simulink model "SR26"  (R2025a)
settings: Solver=FixedStepDiscrete  StartTime=0.0  StopTime=100  FixedStep=0.01  RelTol=1e-3  EnableMultiTasking=on
PreLoadFcn:
  | try, model_open; catch, disp('Error occurred while executing model pre-load callback: model_open.m'); disp('Please assure that the MATLAB working directory is set to the model directory before opening.'); end
InitFcn:
  | try, model_open; catch, end
values from neighbouring files (symbols this model uses):
  dt = 10.0    [SR26.sldd]
undefined symbols (not defined in the file or in its folder): BMSInputProcessing, GCM, raptor_get_safe_string, raptor_xcp_function, RegenEnable, StateCAN, Subsystem, TCEnable
libraries: Utilities x263, Raptor_lib x137, simulink x7, IO x5, APPS_BSPC x4, TorqueCommand x3, Cooling x3, StateMachine x2, DriveSpeed x2, ATCC x2, BrakePressure x2, ThrottlePosition x2
(part 4 of 4)

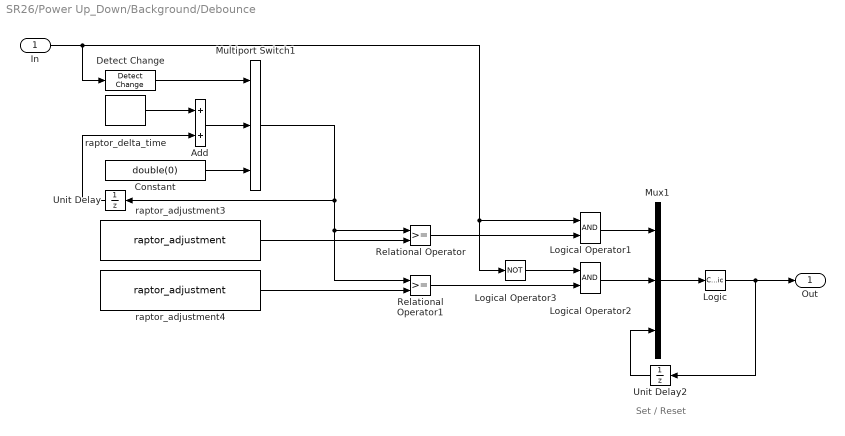
== system SR26/Power Up_Down/Background/Debounce ==
  note: Set / Reset
  In : Inport
  Add : Sum
  Constant : Constant  Value=double(0)
  Detect Change : simulink/Logic and Bit Operations/Detect Change  vinit=0  OutDataTypeStr=boolean
  Logic : CombinatorialLogic  TruthTable=[0;1;0;0;1;1;0;0]
  Logical Operator1 : Logic  AllPortsSameDT=off  OutDataTypeStr=boolean
  Logical Operator2 : Logic  AllPortsSameDT=off  OutDataTypeStr=boolean
  Logical Operator3 : Logic  Operator=NOT  Inputs=1  AllPortsSameDT=off  OutDataTypeStr=boolean
  Multiport Switch1 : MultiPortSwitch  DataPortOrder=Zero-based contiguous  Inputs=2  zeroidx=on  SaturateOnIntegerOverflow=off  InputSameDT=off
  Mux1 : Mux  Inputs=3
  Relational Operator : RelationalOperator  OutDataTypeStr=boolean  InputSameDT=off
  Relational Operator1 : RelationalOperator  OutDataTypeStr=boolean  InputSameDT=off
  Unit Delay : UnitDelay  SampleTime=-1  HasFrameUpgradeWarning=on
  Unit Delay2 : UnitDelay  InitialCondition=1  SampleTime=-1  HasFrameUpgradeWarning=on
  raptor_adjustment3 : Raptor_lib/Data Storage/raptor_adjustment  paramName='KeySwHiTimeThr'  nameSource=Parameter  initValue=0.2  dataType=double  storage=Calibration  calDispType=Number  calEnum={'Active Low', 'Active High'}  calGain=1  calOffset=0  calMax=inf  calMin=-inf  calFormat='-1'  calUnit='sec'  calHelp='State high time threshold'  calAccess=1  calFunction=group  calDispHeaders=off  calColHeaders={'Col1' 'Col2' 'Col3'}  calRowHeaders={'Row1' 'Row2' 'Row3'}
      settings: SourceProductName=Raptor
  raptor_adjustment4 : Raptor_lib/Data Storage/raptor_adjustment  paramName='KeySwLoTimeThr'  nameSource=Parameter  initValue=0.2  dataType=double  storage=Calibration  calDispType=Number  calEnum={'Active Low', 'Active High'}  calGain=1  calOffset=0  calMax=inf  calMin=-inf  calFormat='-1'  calUnit='sec'  calHelp='State low time threshold'  calAccess=1  calFunction=group  calDispHeaders=off  calColHeaders={'Col1' 'Col2' 'Col3'}  calRowHeaders={'Row1' 'Row2' 'Row3'}
      settings: SourceProductName=Raptor
  raptor_delta_time : Raptor_lib/Triggers/raptor_delta_time  unit=seconds
      settings: SourceProductName=Raptor
  Out : Outport  VectorParamsAs1DForOutWhenUnconnected=off
  wires:
  Detect Change/1 -> Multiport Switch1/1
  Logical Operator3/1 -> Logical Operator2/1
  Relational Operator/1 -> Logical Operator1/2
  Logical Operator2/1 -> Mux1/2
  Logical Operator1/1 -> Mux1/1
  Mux1/1 -> Logic/1
  Unit Delay2/1 -> Mux1/3
  In/1 -> Detect Change/1, Logical Operator1/1, Logical Operator3/1
  Multiport Switch1/1 -> Unit Delay/1, Relational Operator/1, Relational Operator1/1
  Add/1 -> Multiport Switch1/2
  Constant/1 -> Multiport Switch1/3
  Relational Operator1/1 -> Logical Operator2/2
  Logic/1 -> Unit Delay2/1, Out/1
  Unit Delay/1 -> Add/2
  raptor_delta_time/1 -> Add/1
  raptor_adjustment4/1 -> Relational Operator1/2
  raptor_adjustment3/1 -> Relational Operator/2

== system SR26/Power Up_Down/Background/Raise Shutdown Event ==
  Trigger : TriggerPort  TriggerType=falling  VariantControl=Variant
  Constant : Constant  Value=boolean(1)
  Function-Call Generator : FunctionCallGenerator  SampleTime=-1
  raptor_data_def : Raptor_lib/Data Storage/raptor_data_def  dataName='FgndTasksStopped'  initValue=0  dataType=boolean  storage=Volatile (RAM)  calVisible=on  calType=Measurement  calDispType=Number  calEnum={'False', 'True'}  calGain=1.0  calOffset=0  calMin=-Inf  calMax=Inf  calFormat='-1'  calUnit='Bool'  calHelp='Boolean indicating foreground tasks stopped'  calAccess=1  calFunction=group  calDispHeaders=off  calColHeaders={'Col1' 'Col2' 'Col3'}  calRowHeaders={'Row1' 'Row2' 'Row3'}
      settings: SourceProductName=Raptor
  raptor_data_write : Raptor_lib/Data Storage/raptor_data_write  dataName='FgndTasksStopped'  dataShape=Scalar  idxSource=Input Port  idxRow=1  idxCol=1
      settings: SourceProductName=Raptor
  raptor_shutdown : Raptor_lib/Triggers/raptor_shutdown  null=0
      settings: SourceProductName=Raptor
  wires:
  Constant/1 -> raptor_data_write/1
  Function-Call Generator/1 -> raptor_shutdown/Trigger

== system SR26/Power Up_Down/Background/Raise Startup Event ==
  Enable : EnablePort
  Trigger : TriggerPort  VariantControl=Variant
  Function-Call Generator : FunctionCallGenerator  SampleTime=-1
  raptor_startup : Raptor_lib/Triggers/raptor_startup  null=0
      settings: SourceProductName=Raptor
  wires:
  Function-Call Generator/1 -> raptor_startup/Trigger

== system SR26/Power Up_Down/Background/Store EEPROM ==
  Trigger : TriggerPort  TriggerType=falling  VariantControl=Variant
  Function-Call Generator : FunctionCallGenerator  SampleTime=-1
  raptor_store_nv : Raptor_lib/Data Storage/raptor_store_nv  null=0
      settings: SourceProductName=Raptor
  wires:
  Function-Call Generator/1 -> raptor_store_nv/Trigger

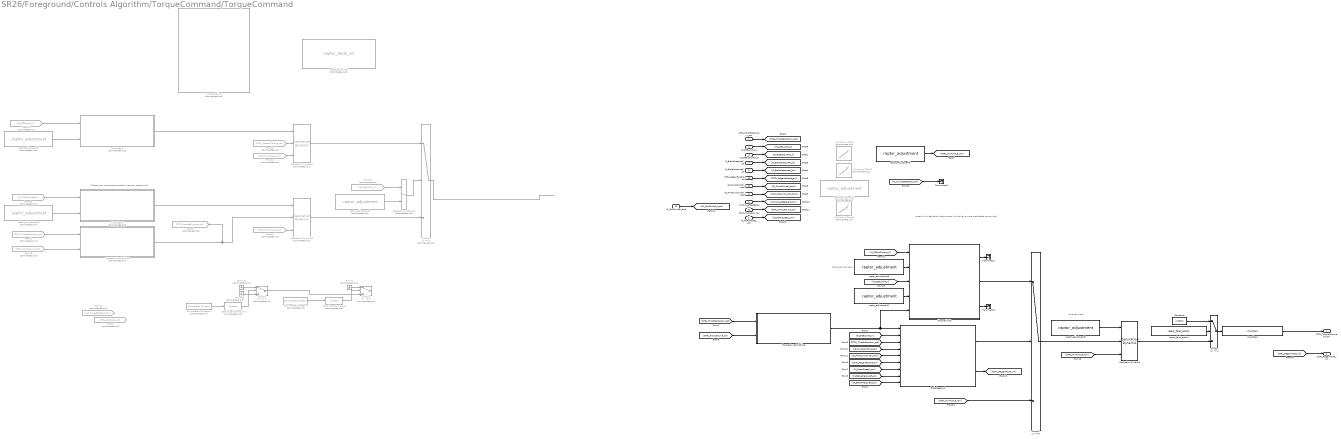
== system SR26/Foreground/Controls Algorithm/TorqueCommand/TorqueCommand ==
  note: current limit (set below legit current limit to have more predictable torque loss)
  note: hard cap here
  note: if there is an overcurrent condition, set new torque limit
  note: these are hard caps
  CTRL_ThrottlePosition_pct : Inport
  IN_DCBusVolt_V : Inport  Port=2
  IN_DCBusCurrent_A : Inport  Port=3
  IN_BrakePressureF_psi : Inport  Port=4
  IN_BrakePressureR_psi : Inport  Port=5
  IN_TorqueFeedback_Nm : Inport  Port=6
  IN_MotorSpeed_rpm : Inport  Port=7
  IO_PwrUpSwitch_bool : Inport  Port=8
  IO_PwrDownSwitch_bool : Inport  Port=9
  IO_CoolSwitch_bool : Inport  Port=10
  CTRL_TorqueCurve_en : Inport  Port=11
  CTRL_RegenEnable_en : Inport  Port=12
  1-D Lookup Table : Lookup_n-D  Commented=on  NumberOfTableDimensions=1  BreakpointsForDimension1=[0;50;100;120;130;140;150;160;170;180;190;200;205;210;215;220;225;230;235;240;245;250;255;260;265;270;275;280;285;290;295;300]  Table=[200;200;200;200;200;200;200;200;200;200;200;200;200;200;200;200;200;200;200;200;200;200;195;190;185;180;175;170;165;160;155;150]  InternalRulePriority=Speed  RndMeth=Simplest
  1-D Lookup Table1 : Lookup_n-D  Commented=on  NumberOfTableDimensions=1  BreakpointsForDimension1=[0;5;10;15;20;25;30;35;40;45;50;55;60;65;70;75;80;85;90;95;100]  Table=[0;3;6;9;12;15;25;35;45;55;65;75;85;95;105;115;135;155;175;195;200]  InternalRulePriority=Speed  RndMeth=Simplest
  1-D Lookup Table2 : Lookup_n-D  Commented=on  NumberOfTableDimensions=1  BreakpointsForDimension1=[0;100;200;205;210;215;220;225;230;235;240;245;250;255;260;265;270;275;280;285;290;300;310;320;330;400]  Table=[0;0;0;25;50;100;125;150;155;160;165;170;175;180;185;190;192;194;196;198;200;200;200;200;200;200]  InternalRulePriority=Speed  RndMeth=Simplest
  BrakeRegen_2 : Subsystem  AncestorBlock=TorqueCommand/BrakeRegen_2
  Constant1 : Constant  Value=uint8(0)
  Data Type Conversion : DataTypeConversion  Commented=on  OutDataTypeStr=boolean  SaturateOnIntegerOverflow=off  RndMeth=Floor
  Data Type Conversion1 : DataTypeConversion  Commented=on  OutDataTypeStr=boolean  SaturateOnIntegerOverflow=off  RndMeth=Floor
  Enumerated Constant : simulink/Sources/Enumerated Constant  Commented=on  OutDataTypeStr=Enum: RegenEnable  Value=RegenEnable.On  SampleTime=inf
  Enumerated Constant1 : simulink/Sources/Enumerated Constant  Commented=on  OutDataTypeStr=Enum: TCEnable  Value=TCEnable.On  SampleTime=inf
  From16 : From  Commented=on  GotoTag=IN_TorqueFeedback_Nm
  From23 : From  Commented=on  GotoTag=IN_DCBusVolt_V
  From24 : From  Commented=on  GotoTag=IN_DCBusVolt_V
  From25 : From  Commented=on  GotoTag=CTRL_AssistedTorque_Nm
  From26 : From  Commented=on  GotoTag=CTRL_MinTorque_Nm
  From27 : From  Commented=on  GotoTag=CTRL_ThrottlePosition_pct
  From28 : From  Commented=on  GotoTag=CTRL_MinTorque_Nm
  From29 : From  Commented=on  GotoTag=CTRL_TorqueCurve_en
  From30 : From  Commented=on  GotoTag=IN_DCBusCurrent_A
  From6 : From  Commented=on  GotoTag=CTRL_SlipRatio_na
  Goto14 : Goto  Commented=on  GotoTag=CTRL_AssistedTorque_Nm
  GreaterThanOrEqual2 : RelationalOperator  Commented=on  Operator=<=  OutDataTypeStr=boolean  RndMeth=Simplest  InputSameDT=off
  Ground : Ground  Commented=on
  Ground1 : Ground  Commented=on
  Ground2 : Ground  Commented=on
  OverMeas : Utilities/OverMeas  sigName='CTRL_TorqueCommand_Nm'  minimum=0  maximum=240
  Saturation Dynamic : simulink/Discontinuities/Saturation Dynamic  OutMin=[]  OutMax=[]  OutDataTypeStr=Inherit: Same as second input  OutDataType=fixdt(1, 16)  OutScaling=2^-10  DoSatur=off
  Saturation Dynamic3 : simulink/Discontinuities/Saturation Dynamic  Commented=on  OutMin=[]  OutMax=[]  OutDataTypeStr=Inherit: Same as second input  OutDataType=fixdt(1, 16)  OutScaling=2^-10  DoSatur=off
  Saturation Dynamic4 : simulink/Discontinuities/Saturation Dynamic  Commented=on  OutMin=[]  OutMax=[]  OutDataTypeStr=Inherit: Same as second input  OutDataType=fixdt(1, 16)  OutScaling=2^-10  DoSatur=off
  Subsystem2 : Subsystem  Commented=on
  Subsystem3 : Subsystem  Commented=on
  Switch : Switch  Criteria=u2 ~= 0  SaturateOnIntegerOverflow=off  InputSameDT=off
  Switch1 : Switch  Commented=on  Criteria=u2 ~= 0  OutDataTypeStr=single  SaturateOnIntegerOverflow=off  InputSameDT=off
  Switch2 : Switch  Criteria=u2 ~= 0  OutDataTypeStr=single  SaturateOnIntegerOverflow=off  InputSameDT=off
  Switch4 : Switch  Commented=on  Criteria=u2 ~= 0  SaturateOnIntegerOverflow=off  InputSameDT=off
  Switch5 : Switch  Commented=on  Criteria=u2 ~= 0  SaturateOnIntegerOverflow=off  InputSameDT=off
  Terminator1 : Terminator
  Terminator2 : Terminator
  Terminator3 : Terminator
  TorqueCeiling : Stateflow chart  Commented=on  TreatAsAtomicUnit=on
  TorqueCurveSwitching : Subsystem
  TorqueCurveSwitching1 : Subsystem  Commented=on
  TorqueLimits : Subsystem  AncestorBlock=TorqueCommand/TorqueLimits
  raptor_adjustment1 : Raptor_lib/Data Storage/raptor_adjustment  paramName='CTRL_DCBusUnderVoltThresh_V'  nameSource=Parameter  initValue=250  dataType=single  storage=Calibration  calDispType=Number  calEnum={'False', 'True'}  calGain=1.0  calOffset=0.0  calMax=378  calMin=-inf  calFormat='-1'  calUnit=''  calHelp=''  calAccess=1  calFunction=raptor_xcp_function(gcb)  calDispHeaders=off  calColHeaders={'Col1' 'Col2' 'Col3'}  calRowHeaders={'Row1' 'Row2' 'Row3'}
      settings: SourceProductName=Raptor
  raptor_adjustment10 : Raptor_lib/Data Storage/raptor_adjustment  Commented=on  paramName='CTRL_CurrentTorqueLimitSetting_na'  nameSource=Parameter  initValue=1  dataType=double  storage=Calibration  calDispType=Number  calEnum={'False', 'True'}  calGain=1.0  calOffset=0.0  calMax=3  calMin=1  calFormat='-1'  calUnit=''  calHelp=''  calAccess=1  calFunction=raptor_xcp_function(gcb)  calDispHeaders=off  calColHeaders={'Col1' 'Col2' 'Col3'}  calRowHeaders={'Row1' 'Row2' 'Row3'}
      settings: SourceProductName=Raptor
  raptor_adjustment11 : Raptor_lib/Data Storage/raptor_adjustment  Commented=on  paramName='CTRL_VoltageTorqueLimitSetting_Nm'  nameSource=Parameter  initValue=1  dataType=double  storage=Calibration  calDispType=Number  calEnum={'False', 'True'}  calGain=1.0  calOffset=0.0  calMax=3  calMin=1  calFormat='-1'  calUnit=''  calHelp=''  calAccess=1  calFunction=raptor_xcp_function(gcb)  calDispHeaders=off  calColHeaders={'Col1' 'Col2' 'Col3'}  calRowHeaders={'Row1' 'Row2' 'Row3'}
      settings: SourceProductName=Raptor
  raptor_adjustment2 : Raptor_lib/Data Storage/raptor_adjustment  paramName='CTRL_MaxTorque'  nameSource=Parameter  initValue=200  dataType=single  storage=Calibration  calDispType=Number  calEnum={'False', 'True'}  calGain=1.0  calOffset=0.0  calMax=230  calMin=0  calFormat='-1'  calUnit=''  calHelp=''  calAccess=1  calFunction=raptor_xcp_function(gcb)  calDispHeaders=off  calColHeaders={'Col1' 'Col2' 'Col3'}  calRowHeaders={'Row1' 'Row2' 'Row3'}
      settings: SourceProductName=Raptor
  raptor_adjustment3 : Raptor_lib/Data Storage/raptor_adjustment  Commented=on  paramName='CTRL_TorqueCurrLim_Nm'  nameSource=Parameter  initValue=100  dataType=single  storage=Calibration  calDispType=Number  calEnum={'False', 'True'}  calGain=1.0  calOffset=0.0  calMax=inf  calMin=-inf  calFormat='-1'  calUnit=''  calHelp=''  calAccess=1  calFunction=raptor_xcp_function(gcb)  calDispHeaders=off  calColHeaders={'Col1' 'Col2' 'Col3'}  calRowHeaders={'Row1' 'Row2' 'Row3'}
      settings: SourceProductName=Raptor
  raptor_adjustment5 : Raptor_lib/Data Storage/raptor_adjustment  paramName='CTRL_MinTorque'  nameSource=Parameter  initValue=-50  dataType=single  storage=Calibration  calDispType=Number  calEnum={'False', 'True'}  calGain=1.0  calOffset=0.0  calMax=230  calMin=-250  calFormat='-1'  calUnit=''  calHelp=''  calAccess=1  calFunction=raptor_xcp_function(gcb)  calDispHeaders=off  calColHeaders={'Col1' 'Col2' 'Col3'}  calRowHeaders={'Row1' 'Row2' 'Row3'}
      settings: SourceProductName=Raptor
  raptor_adjustment8 : Raptor_lib/Data Storage/raptor_adjustment  paramName='CTRL_DCBusOverCurrThresh_A'  nameSource=Parameter  initValue=140  dataType=single  storage=Calibration  calDispType=Number  calEnum={'False', 'True'}  calGain=1.0  calOffset=0.0  calMax=240  calMin=-inf  calFormat='-1'  calUnit=''  calHelp=''  calAccess=1  calFunction=raptor_xcp_function(gcb)  calDispHeaders=off  calColHeaders={'Col1' 'Col2' 'Col3'}  calRowHeaders={'Row1' 'Row2' 'Row3'}
      settings: SourceProductName=Raptor
  raptor_adjustment9 : Raptor_lib/Data Storage/raptor_adjustment  Commented=on  paramName='CTRL_DCBusUnderVoltThresh_V'  nameSource=Parameter  initValue=250  dataType=single  storage=Calibration  calDispType=Number  calEnum={'False', 'True'}  calGain=1.0  calOffset=0.0  calMax=240  calMin=-inf  calFormat='-1'  calUnit=''  calHelp=''  calAccess=1  calFunction=raptor_xcp_function(gcb)  calDispHeaders=off  calColHeaders={'Col1' 'Col2' 'Col3'}  calRowHeaders={'Row1' 'Row2' 'Row3'}
      settings: SourceProductName=Raptor
  raptor_fault_action : Raptor_lib/Faults/raptor_fault_action  actionName='TorqueCmdOverride'  calVisible=on  calAccess=1  calFunction='System | FaultManager | FaultAction'
      settings: SourceProductName=Raptor
  raptor_table_1d3 : Raptor_lib/Table Lookup/raptor_table_1d  Commented=on  dataName='CTRL_TargetSlipRatio_1D'  initValue=[0;764;1528;2293;3057;3822;4586;5350;6114;6880;7643]  dataType=single  storage=Calibration  initValueX=[12;12;12;12;12;12;11.5;11;10.5;10;8]  dataTypeXY=single  storageXY=Calibration  calVisible=on  showTable=on  calGain=1.0  calOffset=0.0  calMax=Inf  calMin=-Inf  calFormat='-1'  calUnit='pct'  calHelp=''  showBreakpoint=on  dataNameX=[]  calGainX=1.0  calOffsetX=0.0  calMaxX=Inf  calMinX=-Inf  calFormatX='-1'  calUnitX='rpm'  calHelpX=''  calAccess=1  calFunction=raptor_xcp_function(gcb)  measureEnable=off  mName=['Data1D_Output']
      settings: SourceProductName=Raptor
  CTRL_TorqueCommand_Nm : Outport
  CTRL_RegenMode_int : Outport  Port=2
  wires:
  TorqueLimits/1(CTRL_TorqueState_en) -> Terminator1/1
  [IN_DCBusVolt_V] -> TorqueLimits/3(IN_DCBusVoltage_V)
  TorqueCurveSwitching/1(Torque) -> BrakeRegen_2/1(TCTorque), TorqueLimits/5(CTRL_TorqueCurve_Nm)
  raptor_adjustment2/1 -> Saturation Dynamic/1
  TorqueLimits/2(CTRL_SafeTorqueCommand_Nm) -> Switch2/1
  [CTRL_MinTorque_Nm] -> Switch2/3
  Saturation Dynamic3/1 -> Switch1/3
  Subsystem2/1(CTRL_CurrentTorqueLimit_Nm) -> Saturation Dynamic3/1
  From24/1 -> Subsystem3/1(IN_DCBusVoltage_V)
  Subsystem3/1(CTRL_CurrentTorqueLimit_Nm) -> Saturation Dynamic4/1
  Saturation Dynamic4/1 -> Switch1/1
  GreaterThanOrEqual2/1 -> Switch1/2
  raptor_adjustment9/1 -> GreaterThanOrEqual2/2
  Switch1/1 -> ?
  From27/1 -> TorqueCurveSwitching1/1(CTRL_ThrottlePosition_pct)
  From29/1 -> TorqueCurveSwitching1/2(CTRL_TorqueCurve_en)
  From30/1 -> Subsystem2/1(IN_DCBusCurrent_A)
  From23/1 -> GreaterThanOrEqual2/1
  From25/1 -> Saturation Dynamic4/2
  From26/1 -> Saturation Dynamic4/3
  From28/1 -> Saturation Dynamic3/3
  raptor_adjustment10/1 -> Subsystem2/2(CTRL_CurrentTorqueSetting_na)
  raptor_adjustment11/1 -> Subsystem3/2(CTRL_VoltageTorqueSetting_na)
  TorqueCurveSwitching1/1(Torque) -> Goto14/1, Saturation Dynamic3/2
  raptor_adjustment8/1 -> TorqueLimits/2(CTRL_DCBusOverCurrThresh_A)
  raptor_adjustment1/1 -> TorqueLimits/4(CTRL_DCBusUnderVoltThresh_V)
  [IN_DCBusCurrent_A] -> TorqueLimits/1(IN_DCBusCurrent_A)
  IO_CoolSwitch_bool/1 -> [IO_CoolSwitch_bool]
  CTRL_TorqueCurve_en/1 -> [CTRL_TorqueCurve_en]
  [CTRL_MinTorque_Nm] -> Saturation Dynamic/3
  raptor_adjustment5/1 -> [CTRL_MinTorque_Nm]
  Ground2/1 -> Switch5/3
  Ground1/1 -> Switch5/1
  Data Type Conversion1/1 -> Switch5/2
  Data Type Conversion/1 -> Switch4/2
  Enumerated Constant1/1 -> Data Type Conversion1/1
  Enumerated Constant/1 -> Data Type Conversion/1
  Switch5/1 -> Switch4/3
  Ground/1 -> Switch4/1
  IN_TorqueFeedback_Nm/1 -> [IN_TorqueFeedback_Nm]
  IO_PwrUpSwitch_bool/1 -> [IO_PwrUpSwitch_bool]
  IO_PwrDownSwitch_bool/1 -> [IO_PwrDownSwitch_bool]
  [CTRL_TorqueCurve_en] -> TorqueCurveSwitching/2(CTRL_TorqueCurve_en)
  CTRL_RegenEnable_en/1 -> [CTRL_RegenEnable_en]
  IN_BrakePressureR_psi/1 -> [IN_BrakePressureR_psi]
  IN_BrakePressureF_psi/1 -> [IN_BrakePressureF_psi]
  CTRL_ThrottlePosition_pct/1 -> [CTRL_ThrottlePosition_pct]
  IN_DCBusCurrent_A/1 -> [IN_DCBusCurrent_A]
  IN_DCBusVolt_V/1 -> [IN_DCBusVolt_V]
  [CTRL_ThrottlePosition_pct] -> TorqueCurveSwitching/1(CTRL_ThrottlePosition_pct)
  Switch2/1 -> Saturation Dynamic/2
  Saturation Dynamic/1 -> Switch/3
  raptor_fault_action/1 -> Switch/2
  OverMeas/1 -> CTRL_TorqueCommand_Nm/1  "CTRL_TorqueCommand_Nm"
  Switch/1 -> OverMeas/1
  Constant1/1 -> Switch/1
  TorqueLimits/3(CTRL_TorqueRedux_Nm) -> Terminator2/1
  BrakeRegen_2/2(CTRL_RegenMode_int) -> [CTRL_RegenMode_int]
  [CTRL_RegenMode_int] -> CTRL_RegenMode_int/1
  [IN_TorqueFeedback_Nm] -> Terminator3/1
  IN_MotorSpeed_rpm/1 -> [IN_MotorSpeed_rpm]
  BrakeRegen_2/1(CTRL_RegenTorque_Nm) -> Switch2/2
  [CTRL_ThrottlePosition_pct] -> BrakeRegen_2/3(CTRL_ThrottlePosition_pct)
  [IN_DCBusVolt_V] -> BrakeRegen_2/2(IN_DCBusVolt_V)
  [IO_PwrUpSwitch_bool] -> BrakeRegen_2/4(IO_PwrUpSwitch_bool)
  [IO_PwrDownSwitch_bool] -> BrakeRegen_2/5(IO_PwrDownSwitch_bool)
  [CTRL_RegenEnable_en] -> BrakeRegen_2/6(CTRL_RegEnable_en)
  [IN_MotorSpeed_rpm] -> BrakeRegen_2/7(IN_MotorSpeed_rpm)
  [IN_BrakePressureF_psi] -> BrakeRegen_2/8(IN_BrakePressureF_psi)
  [IN_BrakePressureR_psi] -> BrakeRegen_2/9(IN_BrakePressureR_psi)

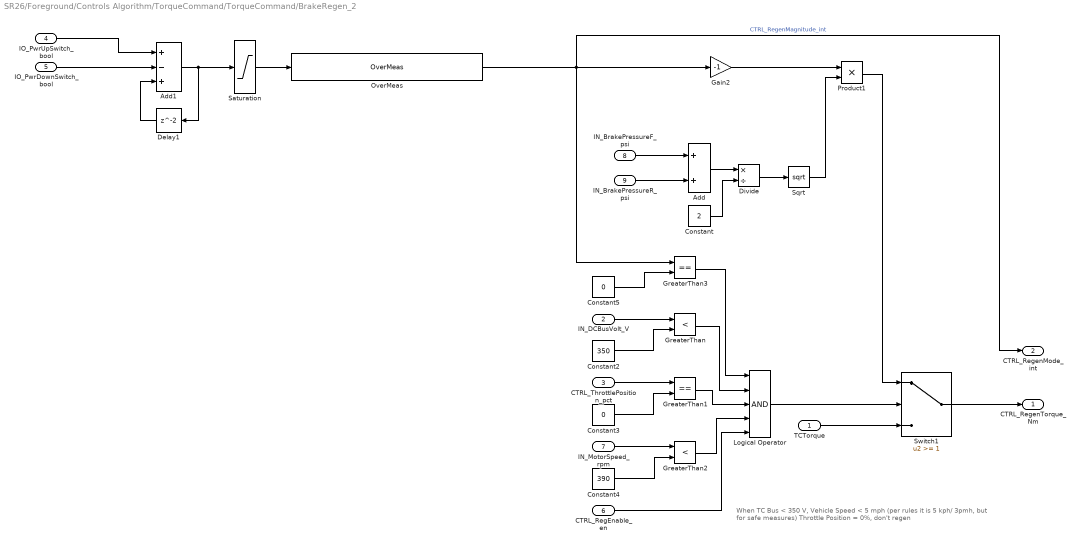
== system SR26/Foreground/Controls Algorithm/TorqueCommand/TorqueCommand/BrakeRegen_2 ==
  note: When TC Bus < 350 V,
      | Vehicle Speed < 5 mph (per rules it is 5 kph/ 3pmh, but for safe measures)
      | Throttle Position = 0%,
      | don't regen
  TCTorque : Inport
  IN_DCBusVolt_V : Inport  Port=2
  CTRL_ThrottlePosition_pct : Inport  Port=3
  IO_PwrUpSwitch_bool : Inport  Port=4
  IO_PwrDownSwitch_bool : Inport  Port=5
  CTRL_RegEnable_en : Inport  Port=6
  IN_MotorSpeed_rpm : Inport  Port=7
  IN_BrakePressureF_psi : Inport  Port=8
  IN_BrakePressureR_psi : Inport  Port=9
  Add : Sum
  Add1 : Sum  Inputs=+-+
  Constant : Constant  Value=2
  Constant2 : Constant  Value=350
  Constant3 : Constant  Value=0
  Constant4 : Constant  Value=390
  Constant5 : Constant  Value=0
  Delay1 : Delay
  Divide : Product  Inputs=*/
  Gain2 : Gain  Gain=-1
  GreaterThan : RelationalOperator  Operator=<  OutDataTypeStr=boolean  RndMeth=Simplest  InputSameDT=off
  GreaterThan1 : RelationalOperator  Operator===  OutDataTypeStr=boolean  RndMeth=Simplest  InputSameDT=off
  GreaterThan2 : RelationalOperator  Operator=<  OutDataTypeStr=boolean  RndMeth=Simplest  InputSameDT=off
  GreaterThan3 : RelationalOperator  Operator===  OutDataTypeStr=boolean  RndMeth=Simplest  InputSameDT=off
  Logical Operator : Logic  Inputs=5  AllPortsSameDT=off  OutDataTypeStr=boolean
  OverMeas : Utilities/OverMeas  sigName='CTRL_RegenMagnitude_int'  minimum=0  maximum=7
  Product1 : Product
  Saturation : Saturate  UpperLimit=7  LowerLimit=0
  Sqrt : Sqrt
  Switch1 : Switch  Threshold=1  SaturateOnIntegerOverflow=off  InputSameDT=off
  CTRL_RegenTorque_Nm : Outport
  CTRL_RegenMode_int : Outport  Port=2
  wires:
  Constant2/1 -> GreaterThan/2
  IN_DCBusVolt_V/1 -> GreaterThan/1
  CTRL_ThrottlePosition_pct/1 -> GreaterThan1/1
  Constant3/1 -> GreaterThan1/2
  IN_MotorSpeed_rpm/1 -> GreaterThan2/1
  Constant4/1 -> GreaterThan2/2
  Logical Operator/1 -> Switch1/2
  IO_PwrUpSwitch_bool/1 -> Add1/1
  IO_PwrDownSwitch_bool/1 -> Add1/2
  Add1/1 -> Saturation/1, Delay1/1
  Delay1/1 -> Add1/3
  Saturation/1 -> OverMeas/1
  TCTorque/1 -> Switch1/3
  OverMeas/1 -> GreaterThan3/1, CTRL_RegenMode_int/1, Gain2/1  "CTRL_RegenMagnitude_int"
  Constant5/1 -> GreaterThan3/2
  GreaterThan3/1 -> Logical Operator/1
  GreaterThan/1 -> Logical Operator/2
  GreaterThan1/1 -> Logical Operator/3
  GreaterThan2/1 -> Logical Operator/4
  CTRL_RegEnable_en/1 -> Logical Operator/5
  Sqrt/1 -> Product1/2
  Divide/1 -> Sqrt/1
  IN_BrakePressureF_psi/1 -> Add/1
  Add/1 -> Divide/1
  Constant/1 -> Divide/2
  IN_BrakePressureR_psi/1 -> Add/2
  Gain2/1 -> Product1/1
  Product1/1 -> Switch1/1
  Switch1/1 -> CTRL_RegenTorque_Nm/1

== system SR26/Foreground/Controls Algorithm/TorqueCommand/TorqueCommand/Subsystem2 ==
  note: decrease at 180A
  note: decrease at 180A
  note: decrease at 150A
  IN_DCBusCurrent_A : Inport
  CTRL_CurrentTorqueSetting_na : Inport  Port=2
  Multiport Switch : MultiPortSwitch  SaturateOnIntegerOverflow=off  InputSameDT=off
  raptor_table_1d1 : Raptor_lib/Table Lookup/raptor_table_1d  dataName='CTRL_CurrentToLimTorqueCmd2_1D'  initValue=[230;230;226;214;194;166;130;86;34;0]  dataType=single  storage=Calibration  initValueX=[0;180;190;200;210;220;230;240;250;260]  dataTypeXY=single  storageXY=Calibration  calVisible=on  showTable=on  calGain=1.0  calOffset=0.0  calMax=Inf  calMin=-Inf  calFormat='-1'  calUnit='Nm'  calHelp=''  showBreakpoint=on  dataNameX=[]  calGainX=1.0  calOffsetX=0.0  calMaxX=Inf  calMinX=-Inf  calFormatX='-1'  calUnitX='A'  calHelpX=''  calAccess=1  calFunction=raptor_xcp_function(gcb)  measureEnable=off  mName=['Data1D_Output']
      settings: SourceProductName=Raptor
  raptor_table_1d2 : Raptor_lib/Table Lookup/raptor_table_1d  dataName='CTRL_CurrentToLimTorqueCmd_1D'  initValue=[230;228;226;222;218;212;206;198;190;180;170;158;146;132;118;102;86;68;50;30;10;0]  dataType=single  storage=Calibration  initValueX=[0;150;155;160;165;170;175;180;185;190;195;200;205;210;215;220;225;230;235;240;245;250]  dataTypeXY=single  storageXY=Calibration  calVisible=on  showTable=on  calGain=1.0  calOffset=0.0  calMax=Inf  calMin=-Inf  calFormat='-1'  calUnit='Nm'  calHelp=''  showBreakpoint=on  dataNameX=[]  calGainX=1.0  calOffsetX=0.0  calMaxX=Inf  calMinX=-Inf  calFormatX='-1'  calUnitX='A'  calHelpX=''  calAccess=1  calFunction=raptor_xcp_function(gcb)  measureEnable=off  mName=['Data1D_Output']
      settings: SourceProductName=Raptor
  raptor_table_1d3 : Raptor_lib/Table Lookup/raptor_table_1d  dataName='CTRL_CurrentToLimTorqueCmd3_1D'  initValue=[230;230;226;214;194;166;130;86;34;0]  dataType=single  storage=Calibration  initValueX=[0;150;160;170;180;190;200;210;220;230]  dataTypeXY=single  storageXY=Calibration  calVisible=on  showTable=on  calGain=1.0  calOffset=0.0  calMax=Inf  calMin=-Inf  calFormat='-1'  calUnit='Nm'  calHelp=''  showBreakpoint=on  dataNameX=[]  calGainX=1.0  calOffsetX=0.0  calMaxX=Inf  calMinX=-Inf  calFormatX='-1'  calUnitX='A'  calHelpX=''  calAccess=1  calFunction=raptor_xcp_function(gcb)  measureEnable=off  mName=['Data1D_Output']
      settings: SourceProductName=Raptor
  CTRL_CurrentTorqueLimit_Nm : Outport
  wires:
  CTRL_CurrentTorqueSetting_na/1 -> Multiport Switch/1
  raptor_table_1d2/1 -> Multiport Switch/2
  raptor_table_1d1/1 -> Multiport Switch/3
  raptor_table_1d3/1 -> Multiport Switch/4
  IN_DCBusCurrent_A/1 -> raptor_table_1d3/1, raptor_table_1d1/1, raptor_table_1d2/1
  Multiport Switch/1 -> CTRL_CurrentTorqueLimit_Nm/1

== system SR26/Foreground/Controls Algorithm/TorqueCommand/TorqueCommand/Subsystem3 ==
  IN_DCBusVoltage_V : Inport
  CTRL_VoltageTorqueSetting_na : Inport  Port=2
  Multiport Switch : MultiPortSwitch  SaturateOnIntegerOverflow=off  InputSameDT=off
  raptor_table_1d1 : Raptor_lib/Table Lookup/raptor_table_1d  dataName='CTRL_VoltageToLimTorqueCmd2_1D'  initValue=[0;0;230;230]  dataType=double  storage=Calibration  initValueX=[0;225;280;378]  dataTypeXY=double  storageXY=Calibration  calVisible=on  showTable=on  calGain=1.0  calOffset=0.0  calMax=Inf  calMin=-Inf  calFormat='-1'  calUnit='Nm'  calHelp=''  showBreakpoint=on  dataNameX=[]  calGainX=1.0  calOffsetX=0.0  calMaxX=Inf  calMinX=-Inf  calFormatX='-1'  calUnitX='V'  calHelpX=''  calAccess=1  calFunction=raptor_xcp_function(gcb)  measureEnable=off  mName=['Data1D_Output']
      settings: SourceProductName=Raptor
  raptor_table_1d2 : Raptor_lib/Table Lookup/raptor_table_1d  dataName='CTRL_VoltageToLimTorqueCmd_1D'  initValue=[0;0;230;230]  dataType=double  storage=Calibration  initValueX=[0;225;280;378]  dataTypeXY=double  storageXY=Calibration  calVisible=on  showTable=on  calGain=1.0  calOffset=0.0  calMax=Inf  calMin=-Inf  calFormat='-1'  calUnit='Nm'  calHelp=''  showBreakpoint=on  dataNameX=[]  calGainX=1.0  calOffsetX=0.0  calMaxX=Inf  calMinX=-Inf  calFormatX='-1'  calUnitX='V'  calHelpX=''  calAccess=1  calFunction=raptor_xcp_function(gcb)  measureEnable=off  mName=['Data1D_Output']
      settings: SourceProductName=Raptor
  raptor_table_1d3 : Raptor_lib/Table Lookup/raptor_table_1d  dataName='CTRL_VoltageToLimTorqueCmd3_1D'  initValue=[0;0;230;230]  dataType=double  storage=Calibration  initValueX=[0;225;280;378]  dataTypeXY=double  storageXY=Calibration  calVisible=on  showTable=on  calGain=1.0  calOffset=0.0  calMax=Inf  calMin=-Inf  calFormat='-1'  calUnit='Nm'  calHelp=''  showBreakpoint=on  dataNameX=[]  calGainX=1.0  calOffsetX=0.0  calMaxX=Inf  calMinX=-Inf  calFormatX='-1'  calUnitX='V'  calHelpX=''  calAccess=1  calFunction=raptor_xcp_function(gcb)  measureEnable=off  mName=['Data1D_Output']
      settings: SourceProductName=Raptor
  CTRL_CurrentTorqueLimit_Nm : Outport
  wires:
  Multiport Switch/1 -> CTRL_CurrentTorqueLimit_Nm/1
  IN_DCBusVoltage_V/1 -> raptor_table_1d2/1, raptor_table_1d3/1, raptor_table_1d1/1
  raptor_table_1d3/1 -> Multiport Switch/4
  raptor_table_1d1/1 -> Multiport Switch/3
  raptor_table_1d2/1 -> Multiport Switch/2
  CTRL_VoltageTorqueSetting_na/1 -> Multiport Switch/1

== system SR26/Foreground/Controls Algorithm/TorqueCommand/TorqueCommand/TorqueCurveSwitching ==
  CTRL_ThrottlePosition_pct : Inport
  CTRL_TorqueCurve_en : Inport  Port=2
  Add : Sum
  Carter : Raptor_lib/Table Lookup/raptor_table_1d  dataName='CTRL_ThrottleToTorqueCmdCarter_1D'  initValue=[0;1;3;6;11;18;25;34;45;57;70;85;101;118;137;158;179;202;227;230;230]  dataType=single  storage=Calibration  initValueX=[0;5;10;15;20;25;30;35;40;45;50;55;60;65;70;75;80;85;90;95;100]  dataTypeXY=single  storageXY=Calibration  calVisible=on  showTable=on  calGain=1.0  calOffset=0.0  calMax=Inf  calMin=-Inf  calFormat='-1'  calUnit='pct'  calHelp=''  showBreakpoint=on  dataNameX=[]  calGainX=1.0  calOffsetX=0.0  calMaxX=Inf  calMinX=-Inf  calFormatX='-1'  calUnitX='Nm'  calHelpX=''  calAccess=1  calFunction=raptor_xcp_function(gcb)  measureEnable=off  mName=['Data1D_Output']
      settings: SourceProductName=Raptor
  Casey : Raptor_lib/Table Lookup/raptor_table_1d  dataName='CTRL_ThrottleToTorqueCmdCasey_1D'  initValue=[0;3;6;9;12;15;25;35;45;55;65;75;85;95;105;115;135;155;175;195;200]  dataType=single  storage=Calibration  initValueX=[0;5;10;15;20;25;30;35;40;45;50;55;60;65;70;75;80;85;90;95;100]  dataTypeXY=single  storageXY=Calibration  calVisible=on  showTable=on  calGain=1.0  calOffset=0.0  calMax=Inf  calMin=-Inf  calFormat='-1'  calUnit='pct'  calHelp=''  showBreakpoint=on  dataNameX=[]  calGainX=1.0  calOffsetX=0.0  calMaxX=Inf  calMinX=-Inf  calFormatX='-1'  calUnitX='Nm'  calHelpX=''  calAccess=1  calFunction=raptor_xcp_function(gcb)  measureEnable=off  mName=['Data1D_Output']
      settings: SourceProductName=Raptor
  Constant : Constant
  Data Type Conversion : DataTypeConversion  OutDataTypeStr=uint8  SaturateOnIntegerOverflow=off  RndMeth=Floor
  Default : Raptor_lib/Table Lookup/raptor_table_1d  dataName='CTRL_ThrottleToTorqueCmdDef_1D'  initValue=[0;3;6;9;12;15;25;35;45;55;65;75;85;95;105;115;135;155;175;195;200]  dataType=single  storage=Calibration  initValueX=[0;5;10;15;20;25;30;35;40;45;50;55;60;65;70;75;80;85;90;95;100]  dataTypeXY=single  storageXY=Calibration  calVisible=on  showTable=on  calGain=1.0  calOffset=0.0  calMax=Inf  calMin=-Inf  calFormat='-1'  calUnit='pct'  calHelp=''  showBreakpoint=on  dataNameX=[]  calGainX=1.0  calOffsetX=0.0  calMaxX=Inf  calMinX=-Inf  calFormatX='-1'  calUnitX='Nm'  calHelpX=''  calAccess=1  calFunction=raptor_xcp_function(gcb)  measureEnable=off  mName=['Data1D_Output']
      settings: SourceProductName=Raptor
  Lim100 : Raptor_lib/Table Lookup/raptor_table_1d  dataName='CTRL_ThrottleToTorqueCmd100_1D'  initValue=[0;8;17;25;33;40;48;55;62;68;74;79;84;88;92;95;97;99;100;100;100]  dataType=single  storage=Calibration  initValueX=[0;5;10;15;20;25;30;35;40;45;50;55;60;65;70;75;80;85;90;95;100]  dataTypeXY=single  storageXY=Calibration  calVisible=on  showTable=on  calGain=1.0  calOffset=0.0  calMax=Inf  calMin=-Inf  calFormat='-1'  calUnit='pct'  calHelp=''  showBreakpoint=on  dataNameX=[]  calGainX=1.0  calOffsetX=0.0  calMaxX=Inf  calMinX=-Inf  calFormatX='-1'  calUnitX='Nm'  calHelpX=''  calAccess=1  calFunction=raptor_xcp_function(gcb)  measureEnable=off  mName=['Data1D_Output']
      settings: SourceProductName=Raptor
  Lim150 : Raptor_lib/Table Lookup/raptor_table_1d  dataName='CTRL_ThrottleToTorqueCmd150_1D'  initValue=[0;8;17;25;33;40;48;55;62;68;74;79;84;88;92;95;97;99;100;100;100]  dataType=single  storage=Calibration  initValueX=[0;5;10;15;20;25;30;35;40;45;50;55;60;65;70;75;80;85;90;95;100]  dataTypeXY=single  storageXY=Calibration  calVisible=on  showTable=on  calGain=1.0  calOffset=0.0  calMax=Inf  calMin=-Inf  calFormat='-1'  calUnit='pct'  calHelp=''  showBreakpoint=on  dataNameX=[]  calGainX=1.0  calOffsetX=0.0  calMaxX=Inf  calMinX=-Inf  calFormatX='-1'  calUnitX='Nm'  calHelpX=''  calAccess=1  calFunction=raptor_xcp_function(gcb)  measureEnable=off  mName=['Data1D_Output']
      settings: SourceProductName=Raptor
  Matt : Raptor_lib/Table Lookup/raptor_table_1d  dataName='CTRL_ThrottleToTorqueCmdMatt_1D'  initValue=[0;3;6;9;12;15;25;35;45;55;65;75;85;95;105;115;135;155;175;195;200]  dataType=single  storage=Calibration  initValueX=[0;5;10;15;20;25;30;35;40;45;50;55;60;65;70;75;80;85;90;95;100]  dataTypeXY=single  storageXY=Calibration  calVisible=on  showTable=on  calGain=1.0  calOffset=0.0  calMax=Inf  calMin=-Inf  calFormat='-1'  calUnit='pct'  calHelp=''  showBreakpoint=on  dataNameX=[]  calGainX=1.0  calOffsetX=0.0  calMaxX=Inf  calMinX=-Inf  calFormatX='-1'  calUnitX='Nm'  calHelpX=''  calAccess=1  calFunction=raptor_xcp_function(gcb)  measureEnable=off  mName=['Data1D_Output']
      settings: SourceProductName=Raptor
  Multiport Switch : MultiPortSwitch  Inputs=7  SaturateOnIntegerOverflow=off  InputSameDT=off
  Noah : Raptor_lib/Table Lookup/raptor_table_1d  dataName='CTRL_ThrottleToTorqueCmdNoah_1D'  initValue=[0;3;6;9;12;15;25;35;45;55;65;75;85;95;105;115;135;155;175;195;200]  dataType=single  storage=Calibration  initValueX=[0;5;10;15;20;25;30;35;40;45;50;55;60;65;70;75;80;85;90;95;100]  dataTypeXY=single  storageXY=Calibration  calVisible=on  showTable=on  calGain=1.0  calOffset=0.0  calMax=Inf  calMin=-Inf  calFormat='-1'  calUnit='pct'  calHelp=''  showBreakpoint=on  dataNameX=[]  calGainX=1.0  calOffsetX=0.0  calMaxX=Inf  calMinX=-Inf  calFormatX='-1'  calUnitX='Nm'  calHelpX=''  calAccess=1  calFunction=raptor_xcp_function(gcb)  measureEnable=off  mName=['Data1D_Output']
      settings: SourceProductName=Raptor
  Torque : Outport
  wires:
  Data Type Conversion/1 -> Add/1
  Constant/1 -> Add/2
  Add/1 -> Multiport Switch/1
  CTRL_TorqueCurve_en/1 -> Data Type Conversion/1
  Multiport Switch/1 -> Torque/1
  Lim100/1 -> Multiport Switch/8
  Lim150/1 -> Multiport Switch/7
  Carter/1 -> Multiport Switch/6
  Noah/1 -> Multiport Switch/5
  Casey/1 -> Multiport Switch/4
  Matt/1 -> Multiport Switch/3
  Default/1 -> Multiport Switch/2
  CTRL_ThrottlePosition_pct/1 -> Matt/1, Casey/1, Noah/1, Carter/1, Lim100/1, Lim150/1, Default/1  "100Nm Limit"

== system SR26/Foreground/Controls Algorithm/TorqueCommand/TorqueCommand/TorqueCurveSwitching1 ==
  CTRL_ThrottlePosition_pct : Inport
  CTRL_TorqueCurve_en : Inport  Port=2
  Add : Sum
  Carter : Raptor_lib/Table Lookup/raptor_table_1d  dataName='CTRL_ThrottleToTorqueCmdCarter_1D'  initValue=[0;1;3;6;11;18;25;34;45;57;70;85;101;118;137;158;179;202;227;230;230]  dataType=single  storage=Calibration  initValueX=[0;5;10;15;20;25;30;35;40;45;50;55;60;65;70;75;80;85;90;95;100]  dataTypeXY=single  storageXY=Calibration  calVisible=on  showTable=on  calGain=1.0  calOffset=0.0  calMax=Inf  calMin=-Inf  calFormat='-1'  calUnit='pct'  calHelp=''  showBreakpoint=on  dataNameX=[]  calGainX=1.0  calOffsetX=0.0  calMaxX=Inf  calMinX=-Inf  calFormatX='-1'  calUnitX='Nm'  calHelpX=''  calAccess=1  calFunction=raptor_xcp_function(gcb)  measureEnable=off  mName=['Data1D_Output']
      settings: SourceProductName=Raptor
  Casey : Raptor_lib/Table Lookup/raptor_table_1d  dataName='CTRL_ThrottleToTorqueCmdCasey_1D'  initValue=[0;3;6;9;12;15;25;35;45;55;65;75;85;95;105;115;135;155;175;195;200]  dataType=single  storage=Calibration  initValueX=[0;5;10;15;20;25;30;35;40;45;50;55;60;65;70;75;80;85;90;95;100]  dataTypeXY=single  storageXY=Calibration  calVisible=on  showTable=on  calGain=1.0  calOffset=0.0  calMax=Inf  calMin=-Inf  calFormat='-1'  calUnit='pct'  calHelp=''  showBreakpoint=on  dataNameX=[]  calGainX=1.0  calOffsetX=0.0  calMaxX=Inf  calMinX=-Inf  calFormatX='-1'  calUnitX='Nm'  calHelpX=''  calAccess=1  calFunction=raptor_xcp_function(gcb)  measureEnable=off  mName=['Data1D_Output']
      settings: SourceProductName=Raptor
  Constant : Constant
  Data Type Conversion : DataTypeConversion  OutDataTypeStr=uint8  SaturateOnIntegerOverflow=off  RndMeth=Floor
  Default : Raptor_lib/Table Lookup/raptor_table_1d  dataName='CTRL_ThrottleToTorqueCmdDef_1D'  initValue=[0;3;6;9;12;15;25;35;45;55;65;75;85;95;105;115;135;155;175;195;200]  dataType=single  storage=Calibration  initValueX=[0;5;10;15;20;25;30;35;40;45;50;55;60;65;70;75;80;85;90;95;100]  dataTypeXY=single  storageXY=Calibration  calVisible=on  showTable=on  calGain=1.0  calOffset=0.0  calMax=Inf  calMin=-Inf  calFormat='-1'  calUnit='pct'  calHelp=''  showBreakpoint=on  dataNameX=[]  calGainX=1.0  calOffsetX=0.0  calMaxX=Inf  calMinX=-Inf  calFormatX='-1'  calUnitX='Nm'  calHelpX=''  calAccess=1  calFunction=raptor_xcp_function(gcb)  measureEnable=off  mName=['Data1D_Output']
      settings: SourceProductName=Raptor
  Lim100 : Raptor_lib/Table Lookup/raptor_table_1d  dataName='CTRL_ThrottleToTorqueCmd100_1D'  initValue=[0;8;17;25;33;40;48;55;62;68;74;79;84;88;92;95;97;99;100;100;100]  dataType=single  storage=Calibration  initValueX=[0;5;10;15;20;25;30;35;40;45;50;55;60;65;70;75;80;85;90;95;100]  dataTypeXY=single  storageXY=Calibration  calVisible=on  showTable=on  calGain=1.0  calOffset=0.0  calMax=Inf  calMin=-Inf  calFormat='-1'  calUnit='pct'  calHelp=''  showBreakpoint=on  dataNameX=[]  calGainX=1.0  calOffsetX=0.0  calMaxX=Inf  calMinX=-Inf  calFormatX='-1'  calUnitX='Nm'  calHelpX=''  calAccess=1  calFunction=raptor_xcp_function(gcb)  measureEnable=off  mName=['Data1D_Output']
      settings: SourceProductName=Raptor
  Lim150 : Raptor_lib/Table Lookup/raptor_table_1d  dataName='CTRL_ThrottleToTorqueCmd150_1D'  initValue=[0;8;17;25;33;40;48;55;62;68;74;79;84;88;92;95;97;99;100;100;100]  dataType=single  storage=Calibration  initValueX=[0;5;10;15;20;25;30;35;40;45;50;55;60;65;70;75;80;85;90;95;100]  dataTypeXY=single  storageXY=Calibration  calVisible=on  showTable=on  calGain=1.0  calOffset=0.0  calMax=Inf  calMin=-Inf  calFormat='-1'  calUnit='pct'  calHelp=''  showBreakpoint=on  dataNameX=[]  calGainX=1.0  calOffsetX=0.0  calMaxX=Inf  calMinX=-Inf  calFormatX='-1'  calUnitX='Nm'  calHelpX=''  calAccess=1  calFunction=raptor_xcp_function(gcb)  measureEnable=off  mName=['Data1D_Output']
      settings: SourceProductName=Raptor
  Matt : Raptor_lib/Table Lookup/raptor_table_1d  dataName='CTRL_ThrottleToTorqueCmdMatt_1D'  initValue=[0;3;6;9;12;15;25;35;45;55;65;75;85;95;105;115;135;155;175;195;200]  dataType=single  storage=Calibration  initValueX=[0;5;10;15;20;25;30;35;40;45;50;55;60;65;70;75;80;85;90;95;100]  dataTypeXY=single  storageXY=Calibration  calVisible=on  showTable=on  calGain=1.0  calOffset=0.0  calMax=Inf  calMin=-Inf  calFormat='-1'  calUnit='pct'  calHelp=''  showBreakpoint=on  dataNameX=[]  calGainX=1.0  calOffsetX=0.0  calMaxX=Inf  calMinX=-Inf  calFormatX='-1'  calUnitX='Nm'  calHelpX=''  calAccess=1  calFunction=raptor_xcp_function(gcb)  measureEnable=off  mName=['Data1D_Output']
      settings: SourceProductName=Raptor
  Multiport Switch : MultiPortSwitch  Inputs=7  SaturateOnIntegerOverflow=off  InputSameDT=off
  Noah : Raptor_lib/Table Lookup/raptor_table_1d  dataName='CTRL_ThrottleToTorqueCmdNoah_1D'  initValue=[0;3;6;9;12;15;25;35;45;55;65;75;85;95;105;115;135;155;175;195;200]  dataType=single  storage=Calibration  initValueX=[0;5;10;15;20;25;30;35;40;45;50;55;60;65;70;75;80;85;90;95;100]  dataTypeXY=single  storageXY=Calibration  calVisible=on  showTable=on  calGain=1.0  calOffset=0.0  calMax=Inf  calMin=-Inf  calFormat='-1'  calUnit='pct'  calHelp=''  showBreakpoint=on  dataNameX=[]  calGainX=1.0  calOffsetX=0.0  calMaxX=Inf  calMinX=-Inf  calFormatX='-1'  calUnitX='Nm'  calHelpX=''  calAccess=1  calFunction=raptor_xcp_function(gcb)  measureEnable=off  mName=['Data1D_Output']
      settings: SourceProductName=Raptor
  Torque : Outport
  wires:
  CTRL_ThrottlePosition_pct/1 -> Lim150/1, Lim100/1, Carter/1, Noah/1, Casey/1, Matt/1, Default/1  "100Nm Limit"
  Default/1 -> Multiport Switch/2
  Matt/1 -> Multiport Switch/3
  Casey/1 -> Multiport Switch/4
  Noah/1 -> Multiport Switch/5
  Carter/1 -> Multiport Switch/6
  Lim150/1 -> Multiport Switch/7
  Lim100/1 -> Multiport Switch/8
  Multiport Switch/1 -> Torque/1
  CTRL_TorqueCurve_en/1 -> Data Type Conversion/1
  Add/1 -> Multiport Switch/1
  Constant/1 -> Add/2
  Data Type Conversion/1 -> Add/1

== system SR26/Foreground/Controls Algorithm/TorqueCommand/TorqueCommand/TorqueLimits ==
  IN_DCBusCurrent_A : Inport
  CTRL_DCBusOverCurrThresh_A : Inport  Port=2
  IN_DCBusVoltage_V : Inport  Port=3
  CTRL_DCBusUnderVoltThresh_V : Inport  Port=4
  CTRL_TorqueCurve_Nm : Inport  Port=5
  Ground : Ground
  Max : MinMax  Function=max  Inputs=2
  OCRedux : TorqueCommand/OCRedux  SystemSampleTime=-1  VariantActivationTime=update diagram  EmptyChoice=off  PassThrough=off  PassThroughVariantControl=(default)  EmptyChoiceVariantControl=(default)  AllowFlexibleInterface=on  Latency=0  AutoFrameSizeCalculation=off
  OverMeas : Utilities/OverMeas  sigName='CTRL_SafeTorqueCommand_Nm'  minimum=-inf  maximum=inf
  OverMeas1 : Utilities/OverMeas  sigName='CTRL_TorqueRedux_Nm'  minimum=-inf  maximum=inf
  Subtract : Sum  Inputs=-+
  UVRedux : TorqueCommand/UVRedux  SystemSampleTime=-1  VariantActivationTime=update diagram  EmptyChoice=off  PassThrough=off  PassThroughVariantControl=(default)  EmptyChoiceVariantControl=(default)  AllowFlexibleInterface=on  Latency=0  AutoFrameSizeCalculation=off
  CTRL_TorqueState_en : Outport
  CTRL_SafeTorqueCommand_Nm : Outport  Port=2
  CTRL_TorqueRedux_Nm : Outport  Port=3
  wires:
  OCRedux/1 -> Max/1
  IN_DCBusCurrent_A/1 -> OCRedux/1
  CTRL_DCBusOverCurrThresh_A/1 -> OCRedux/2
  Max/1 -> OverMeas1/1, Subtract/1
  CTRL_TorqueCurve_Nm/1 -> Subtract/2
  Subtract/1 -> OverMeas/1
  OverMeas/1 -> CTRL_SafeTorqueCommand_Nm/1  "CTRL_SafeTorqueCommand_Nm"
  UVRedux/1 -> Max/2
  IN_DCBusVoltage_V/1 -> UVRedux/1
  CTRL_DCBusUnderVoltThresh_V/1 -> UVRedux/2
  Ground/1 -> CTRL_TorqueState_en/1
  OverMeas1/1 -> CTRL_TorqueRedux_Nm/1  "CTRL_TorqueRedux_Nm"

== stateflow chart SR26/Foreground/Controls Algorithm/TorqueCommand/TorqueCommand/TorqueCeiling ==
  state Default
    en:
    State = TorqueCeiling.NA;
    Torque = 230;
  state UnderVoltage
    en:
    State = TorqueCeiling.UnderVoltage;
    state UnderVoltInit
      en:
      Torque = 100;
    state UnderVolt3
      en:
      Torque = 50;
    state UnderVolt2
      en:
      Torque = 50;
    (default) -> UnderVoltInit
    UnderVoltInit -> UnderVolt3 : [DCBusVolts >= UnderVoltageThreshold]
    UnderVolt3 -> UnderVolt2 : [DCBusVolts >= UnderVoltageThreshold]
  state OverCurrent1
    en:
    State = TorqueCeiling.OverCurr;
    state OverCurrInit
      en:
      Torque = 100;
    state OverCurr2
      en:
      Torque = 70;
    state OverCurr3
      en:
      Torque = 50;
    (default) -> OverCurrInit
    OverCurrInit -> OverCurr2 : [DCBusCurrent >= OverCurrentThreshold]
    OverCurr2 -> OverCurr3 : [DCBusCurrent >= OverCurrentThreshold]
  (default) -> Default
  Default -> (junction 31) [order 2] : [DCBusVolts >= UnderVoltageThreshold]
  Default -> (junction 18) [order 1] : [DCBusCurrent >= OverCurrentThreshold]
  (junction 31) -> UnderVoltage
  (junction 18) -> OverCurrent1
  (junction 34) -> Default
  UnderVoltage -> (junction 34) : [ThrottlePosition <= 50]
  OverCurrent1 -> (junction 34) : [ThrottlePosition <= 50]
  data: DCBusVolts input; DCBusCurrent input; ThrottlePosition input; UnderVoltageThreshold input; OverCurrentThreshold input; State output; Torque output
